simulink model "guidance_law"  (R2018a)
settings: Solver=VariableStepAuto  StartTime=0.0  StopTime=0.95  RelTol=1e-3
values from neighbouring files (symbols this model uses):
  cd = 0.5    [guidance_law_param.m]
  first_term_coeff = 2+sqrt(4+N+2*M)    [guidance_law_param.m]
  g = 9.81    [guidance_law_param.m]
  init_lambda = -atan(3/4)    [guidance_law_param.m]
  init_pos = [0,3]    [guidance_law_param.m]
  init_vel = 2.5    [guidance_law_param.m]
  lambda_desired = -(0/180)*pi    (= 0)    [guidance_law_param.m]
  M = 8    [guidance_law_param.m]
  mass = 5    [guidance_law_param.m]
  rho = 1.293    [guidance_law_param.m]
  S = 0    [guidance_law_param.m]
  target_pos = [4,0]    [guidance_law_param.m]
undefined symbols (not defined in the file or in its folder): magnitude
settings Model: Creator=Lee  LastModifiedBy=Lee

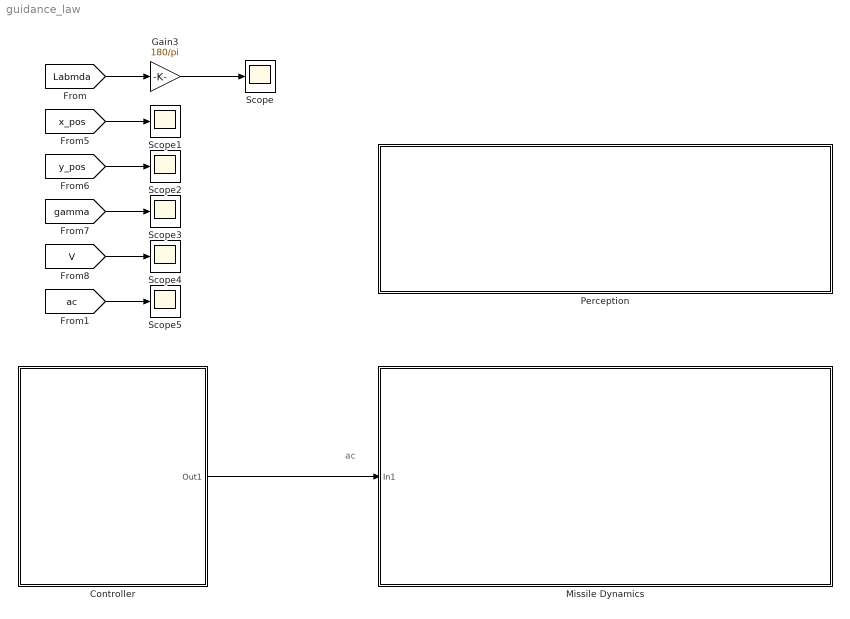
== system guidance_law ==
  note: ac
  Controller : Subsystem
  Gain3 : Gain  Gain=180/pi
  Missile Dynamics : Subsystem
  Perception : Subsystem
  Scope{,1..5} (6 alike) : Scope
  wires:
  Controller/1(Out1) -> Missile Dynamics/1(In1)
  [x_pos] -> Scope1/1
  [y_pos] -> Scope2/1
  [gamma] -> Scope3/1
  [V] -> Scope4/1
  [ac] -> Scope5/1
  [Labmda] -> Gain3/1
  Gain3/1 -> Scope/1

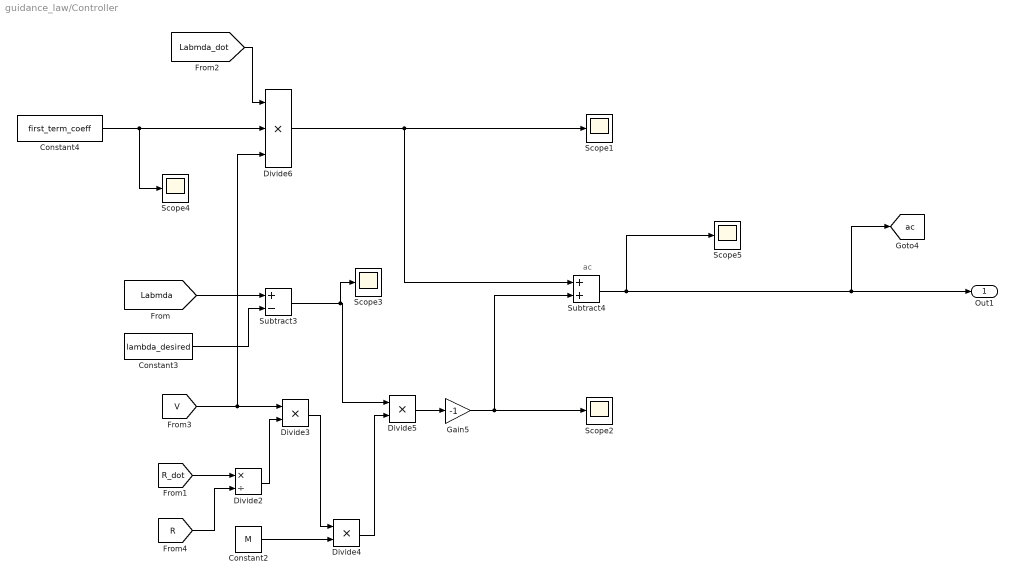
== system guidance_law/Controller ==
  note: ac
  Constant2 : Constant  Value=M
  Constant3 : Constant  Value=lambda_desired
  Constant4 : Constant  Value=first_term_coeff
  Divide2 : Product  Inputs=*/
  Divide3 : Product  Inputs=**
  Divide4 : Product  Inputs=**
  Divide5 : Product  Inputs=**
  Divide6 : Product  Inputs=***
  Gain5 : Gain  Gain=-1
  Scope{1..5} (5 alike) : Scope
  Subtract3 : Sum  Inputs=+-
  Subtract4 : Sum
  Out1 : Outport
  tag scope: ac=global
  wires:
  Divide5/1 -> Gain5/1
  Subtract4/1 -> [ac], Out1/1, Scope5/1
  Constant3/1 -> Subtract3/2
  Subtract3/1 -> Scope3/1, Divide5/1
  [R_dot] -> Divide2/1
  [R] -> Divide2/2
  Divide3/1 -> Divide4/1
  [V] -> Divide6/3, Divide3/1
  [Labmda_dot] -> Divide6/1
  Divide6/1 -> Subtract4/1, Scope1/1
  [Labmda] -> Subtract3/1
  Divide4/1 -> Divide5/2
  Gain5/1 -> Scope2/1, Subtract4/2
  Divide2/1 -> Divide3/2
  Constant4/1 -> Scope4/1, Divide6/2
  Constant2/1 -> Divide4/2

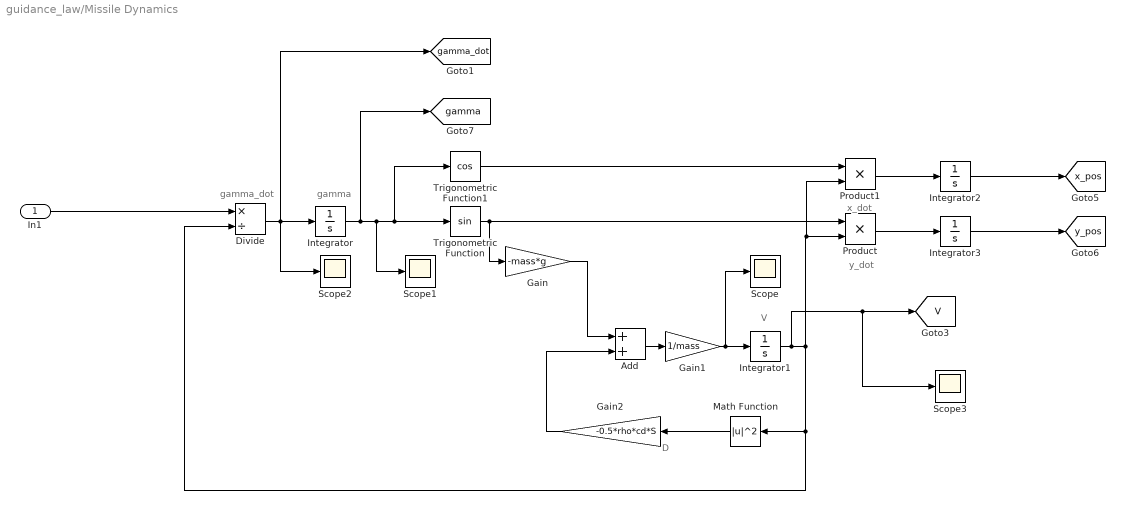
== system guidance_law/Missile Dynamics ==
  note: V
  note: D
  note: gamma_dot
  note: x_dot
  note: y_dot
  note: gamma
  In1 : Inport
  Add : Sum
  Divide : Product  Inputs=*/
  Gain : Gain  Gain=-mass*g
  Gain1 : Gain  Gain=1/mass
  Gain2 : Gain  Gain=-0.5*rho*cd*S
  Integrator : Integrator
  Integrator1 : Integrator  InitialCondition=init_vel
  Integrator2 : Integrator  InitialCondition=init_pos(1)
  Integrator3 : Integrator  InitialCondition=init_pos(2)
  Math Function : Math  Operator=magnitude^2  SaturateOnIntegerOverflow=on
  Product : Product
  Product1 : Product
  Scope{,1..3} (4 alike) : Scope
  Trigonometric Function : Trigonometry
  Trigonometric Function1 : Trigonometry  Operator=cos
  tag scope: V=global, gamma=global, gamma_dot=global, x_pos=global, y_pos=global
  wires:
  Integrator1/1 -> Scope3/1, [V], Product1/2, Product/2, Divide/2, Math Function/1
  Product1/1 -> Integrator2/1
  Divide/1 -> [gamma_dot], Scope2/1, Integrator/1
  Integrator2/1 -> [x_pos]
  Trigonometric Function/1 -> Product/1, Gain/1
  Gain/1 -> Add/1
  Integrator/1 -> [gamma], Scope1/1, Trigonometric Function1/1, Trigonometric Function/1
  Math Function/1 -> Gain2/1
  Gain2/1 -> Add/2
  Integrator3/1 -> [y_pos]
  Trigonometric Function1/1 -> Product1/1
  Gain1/1 -> Scope/1, Integrator1/1
  Product/1 -> Integrator3/1
  Add/1 -> Gain1/1
  In1/1 -> Divide/1

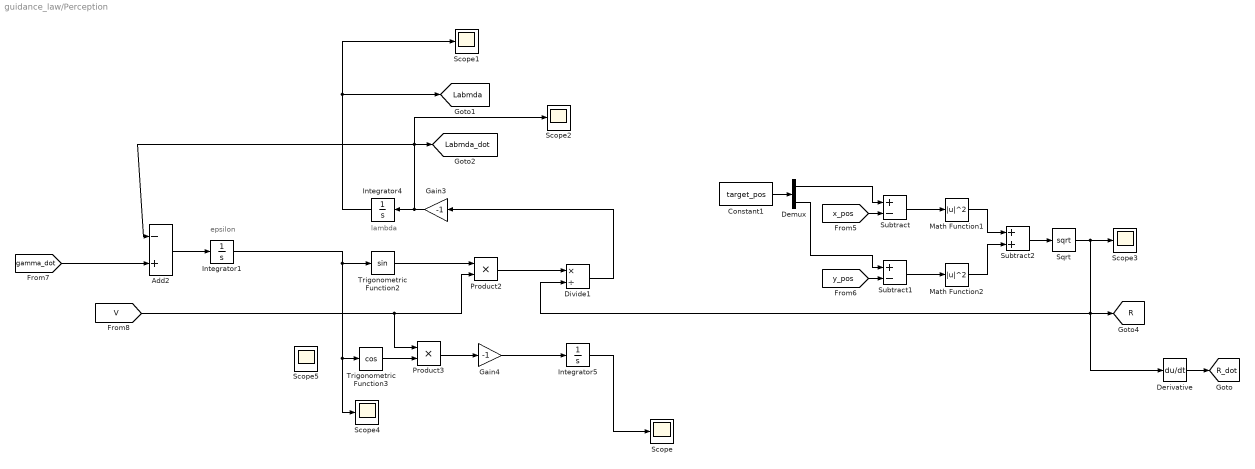
== system guidance_law/Perception ==
  note: lambda
  note: epsilon
  Add2 : Sum  Inputs=-+
  Constant1 : Constant  Value=target_pos
  Demux : Demux  Outputs=2
  Derivative : Derivative
  Divide1 : Product  Inputs=*/
  Gain3 : Gain  Gain=-1
  Gain4 : Gain  Gain=-1
  Integrator1 : Integrator  InitialCondition=-init_lambda
  Integrator4 : Integrator  InitialCondition=init_lambda
  Integrator5 : Integrator  InitialCondition=5000
  Math Function1 : Math  Operator=magnitude^2  SaturateOnIntegerOverflow=on
  Math Function2 : Math  Operator=magnitude^2  SaturateOnIntegerOverflow=on
  Product2 : Product
  Product3 : Product
  Scope{,1..5} (6 alike) : Scope
  Sqrt : Sqrt  SaturateOnIntegerOverflow=on
  Subtract : Sum  Inputs=+-
  Subtract1 : Sum  Inputs=+-
  Subtract2 : Sum
  Trigonometric Function2 : Trigonometry
  Trigonometric Function3 : Trigonometry  Operator=cos
  tag scope: Labmda=global, Labmda_dot=global, R=global, R_dot=global
  wires:
  [x_pos] -> Subtract/2
  [V] -> Product3/1, Product2/2
  Gain3/1 -> Integrator4/1, Add2/1, Scope2/1, [Labmda_dot]
  Math Function1/1 -> Subtract2/1
  Product2/1 -> Divide1/1
  [y_pos] -> Subtract1/2
  Demux/1 -> Subtract/1
  Trigonometric Function2/1 -> Product2/1
  Constant1/1 -> Demux/1
  Subtract2/1 -> Sqrt/1
  Integrator1/1 -> Scope4/1, Trigonometric Function3/1, Trigonometric Function2/1
  Integrator4/1 -> Scope1/1, [Labmda]
  Subtract1/1 -> Math Function2/1
  Divide1/1 -> Gain3/1
  Gain4/1 -> Integrator5/1
  Integrator5/1 -> Scope/1
  Product3/1 -> Gain4/1
  Demux/2 -> Subtract1/1
  Math Function2/1 -> Subtract2/2
  Subtract/1 -> Math Function1/1
  Trigonometric Function3/1 -> Product3/2
  Sqrt/1 -> Divide1/2, [R], Derivative/1, Scope3/1
  Derivative/1 -> [R_dot]
  [gamma_dot] -> Add2/2
  Add2/1 -> Integrator1/1
